simulink model "SFRM_with_UFLS_simulink"  (R2023b)
settings: Solver=FixedStepAuto  StartTime=0.0  StopTime=10.0  FixedStep=0.001  RelTol=1e-3
values from neighbouring files (symbols this model uses):
  D = 1    [SFRM_with_UFLS_script.m]
  f_rated = 50    [SFRM_with_UFLS_script.m]
  FH = 0.3    [SFRM_with_UFLS_script.m]
  fLIM = 47.5    [SFRM_with_UFLS_script.m]
  fthr_instance = [49.0  48.8  48.6  48.4  48.2  48.0]    [SFRM_with_UFLS_script.m]
  H = 4    [SFRM_with_UFLS_script.m]
  K = -0.70    (= -0.7)    [SFRM_with_UFLS_script.m]
  KM = 0.95    [SFRM_with_UFLS_script.m]
  Mthr_instance = [2.0   1.80  1.60  1.40  1.20  1.00]    [SFRM_with_UFLS_script.m]
  R = 0.05    [SFRM_with_UFLS_script.m]
  TR = 8    [SFRM_with_UFLS_script.m]
  UFLS_stages = [0.10  0.10  0.10  0.10  0.10  0.10]    [SFRM_with_UFLS_script.m]
  UFLS_type = 3    [SFRM_with_UFLS_script.m]
libraries: simulink x4
settings Model: Creator=urbanr  LastModifiedBy=urban
settings DebuggingCC: ParameterPrecisionLossMsg=none

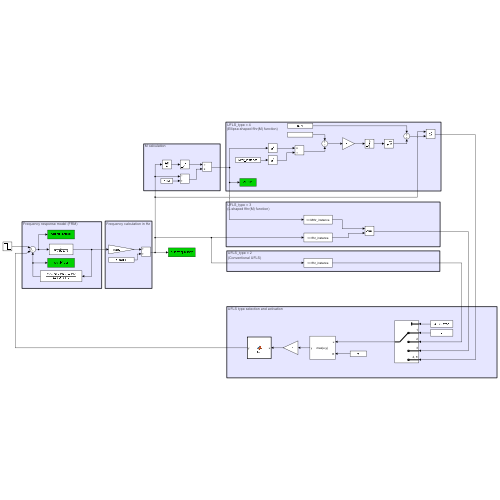
[thumbnail: Simulink's stored preview of the top-level diagram]
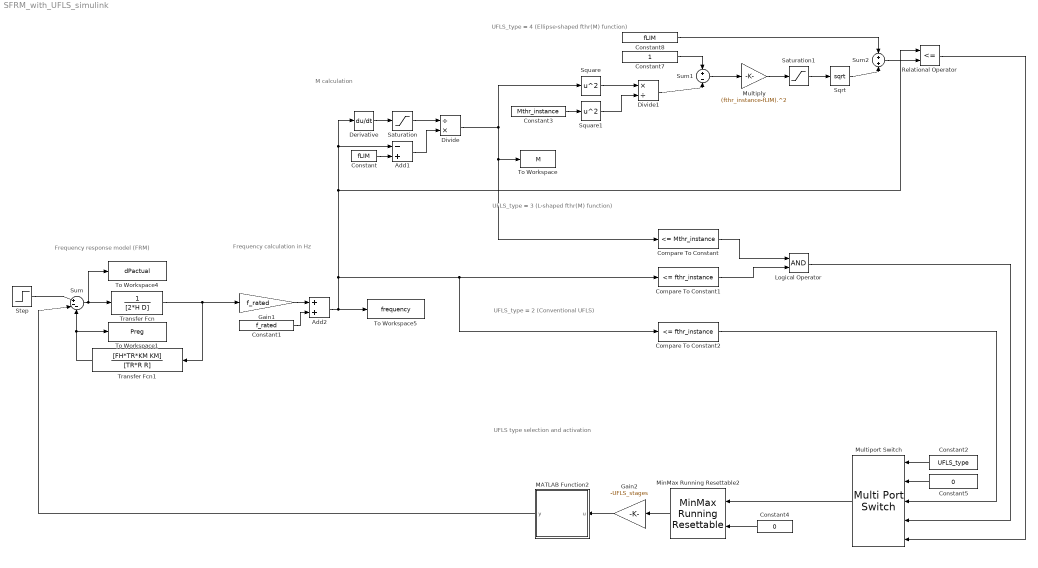
== system SFRM_with_UFLS_simulink ==
  note: UFLS_type = 2
      | (Conventional UFLS)
  note: UFLS_type = 3
      | (L-shaped fthr(M) function)
  note: UFLS type selection and activation
  note: UFLS_type = 4
      | (Ellipse-shaped fthr(M) function)
  note: Frequency calculation in Hz
  note: Frequency response model (FRM)
  note: M calculation
  Add1 : Sum  Inputs=-+
  Add2 : Sum
  Compare To Constant : simulink/Logic and Bit Operations/Compare To Constant  relop=<=  const=Mthr_instance  OutDataTypeStr=boolean
  Compare To Constant1 : simulink/Logic and Bit Operations/Compare To Constant  relop=<=  const=fthr_instance  OutDataTypeStr=boolean
  Compare To Constant2 : simulink/Logic and Bit Operations/Compare To Constant  relop=<=  const=fthr_instance  OutDataTypeStr=boolean
  Constant : Constant  Value=fLIM
  Constant1 : Constant  Value=f_rated
  Constant2 : Constant  Value=UFLS_type
  Constant3 : Constant  Value=Mthr_instance
  Constant4 : Constant  Value=0
  Constant5 : Constant  Value=0
  Constant7 : Constant
  Constant8 : Constant  Value=fLIM
  Derivative : Derivative
  Divide : Product  Inputs=/*
  Divide1 : Product  Inputs=*/
  Gain1 : Gain  Gain=f_rated
  Gain2 : Gain  Gain=-UFLS_stages
  Logical Operator : Logic  AllPortsSameDT=off  OutDataTypeStr=boolean
  MATLAB Function2 : MATLAB Function  TreatAsAtomicUnit=on
  MinMax Running Resettable2 : simulink/Math Operations/MinMax Running Resettable  Function=max  vinit=0.0
  Multiply : Gain  Gain=(fthr_instance-fLIM).^2
  Multiport Switch : MultiPortSwitch  Inputs=4  SaturateOnIntegerOverflow=off  InputSameDT=off
  Relational Operator : RelationalOperator  Operator=<=  OutDataTypeStr=boolean  RndMeth=Simplest  InputSameDT=off
  Saturation : Saturate  UpperLimit=-1e-15  LowerLimit=-1e+9
  Saturation1 : Saturate  UpperLimit=1e9  LowerLimit=0
  Sqrt : Sqrt
  Square : Math  Operator=square
  Square1 : Math  Operator=square
  Step : Step  After=K  SampleTime=0
  Sum : Sum  Inputs=|+--
  Sum1 : Sum  Inputs=+-
  Sum2 : Sum
  To Workspace : ToWorkspace  VariableName=M  SampleTime=-1
      settings: Save2DSignal=2-D array (concatenate along first dimension)
  To Workspace1 : ToWorkspace  VariableName=Preg  SampleTime=-1
  To Workspace4 : ToWorkspace  VariableName=dPactual  SampleTime=-1
  To Workspace5 : ToWorkspace  VariableName=frequency  SampleTime=-1
  Transfer Fcn : TransferFcn  Denominator=[2*H D]
  Transfer Fcn1 : TransferFcn  Numerator=[FH*TR*KM KM]  Denominator=[TR*R R]
  wires:
  Constant1/1 -> Add2/2
  Transfer Fcn/1 -> Transfer Fcn1/1, Gain1/1
  Transfer Fcn1/1 -> Sum/3, To Workspace1/1
  Sum/1 -> To Workspace4/1, Transfer Fcn/1
  Gain1/1 -> Add2/1
  Add2/1 -> Derivative/1, Add1/1, Relational Operator/1, Compare To Constant2/1, Compare To Constant1/1, To Workspace5/1
  Add1/1 -> Divide/2
  Saturation/1 -> Divide/1
  Constant/1 -> Add1/2
  Step/1 -> Sum/1
  Compare To Constant/1 -> Logical Operator/1
  Compare To Constant1/1 -> Logical Operator/2
  Derivative/1 -> Saturation/1
  Divide/1 -> Compare To Constant/1, To Workspace/1, Square/1
  Constant3/1 -> Square1/1
  Square/1 -> Divide1/1
  Square1/1 -> Divide1/2
  Constant7/1 -> Sum1/1
  Divide1/1 -> Sum1/2
  Sum1/1 -> Multiply/1
  Sum2/1 -> Relational Operator/2
  Sqrt/1 -> Sum2/2
  Constant8/1 -> Sum2/1
  Multiply/1 -> Saturation1/1
  Saturation1/1 -> Sqrt/1
  Constant2/1 -> Multiport Switch/1
  Multiport Switch/1 -> MinMax Running Resettable2/1
  Constant4/1 -> MinMax Running Resettable2/2
  MinMax Running Resettable2/1 -> Gain2/1
  Gain2/1 -> MATLAB Function2/1(u)
  MATLAB Function2/1(y) -> Sum/2
  Constant5/1 -> Multiport Switch/2
  Compare To Constant2/1 -> Multiport Switch/3
  Logical Operator/1 -> Multiport Switch/4
  Relational Operator/1 -> Multiport Switch/5

== matlab function SFRM_with_UFLS_simulink/MATLAB Function2 ==
  data: u input; y output
function y = fcn(u)
    y = sum(u);
